simulink model "real_UIO_EEG_2021_03_03_01"  (R2019b)
settings: Solver=FixedStepAuto  StartTime=0.0  StopTime=180  FixedStep=0.01  RelTol=1e-3
values from neighbouring files (symbols this model uses):
  Am = double(subs(Am_sys,{ep,Lx},{0.1,1-2*j}))    [DAC_UIO_Comp.m]    (also in UIO_adaptive_example_EEG_Balas_2ch.m = [0 1;-5 -4]; UIO_adaptive_example_alternative_EEG_ch6.m = ss_c.A; UIO_alternative_2021_01_26.m = Am-.1*eye(2); UIO_alternative_PAPER_2021_02_17.m = [0 1;-1 -1])
  B = [0;1]    [DAC_UIO_Comp.m]    (also in UIO_adaptive_example_EEG_Balas_2ch.m; UIO_adaptive_example_alternative_EEG_ch6.m = ones(opt_order,1); UIO_alternative_2021_01_26.m; UIO_alternative_PAPER_2021_02_17.m = [1;0;-1])
  C = double(subs(C_sym,{ep},{0.1}))    [DAC_UIO_Comp.m]    (also in UIO_adaptive_example.m = [1 0 0 0 0;0 0 0 1 0; 0 0 0 0 1]; UIO_adaptive_example_2.m = [1 0 0 0;0 1 0 0]; UIO_adaptive_example_EEG_Balas_2ch.m = [1, epsilon]; UIO_adaptive_example_alternative_EEG_ch6.m = ss_c.C)
  Fu = mats    [UIO_adaptive_example_alternative_EEG_ch6.m]    (also in UIO_alternative_2021_01_26.m = [0 1 ;-25 0]; UIO_alternative_PAPER_2021_02_17.m = [0,0,0,0, 0;0 0 1 0 0;0 -25 0 0 0;0 0 0 0 1;0 0 0 -144 0]; UIO_alternative_PAPER_2021_03_01.m = [0 1 0 0;-25 0 0 0;0 0 0 1;0 0 -144 0]; UIO_alternative_PAPER_2021_03_02.m = [0 1 0 0;-25 0 0 0;0 0 0 1;0 0 -144 0])
  gamma_e = 1    [DAC_UIO_Comp.m]    (also in UIO_adaptive_example_EEG_Balas_2ch.m; UIO_adaptive_example_alternative_EEG_ch6.m = .0001*ones(length(Am),1); UIO_alternative_2021_01_26.m = 0.001; UIO_alternative_PAPER_2021_02_17.m = 0.0001)
  K1 = Klqr(1:length(Am),:)    [UIO_adaptive_example_alternative_EEG_ch6.m]    (also in UIO_alternative_PAPER_2021_03_02.m = Kout3(1:length(Am),:))
  K2 = Klqr(length(Am)+1:end,:)    [UIO_adaptive_example_alternative_EEG_ch6.m]    (also in UIO_alternative_PAPER_2021_03_02.m = Kout3(length(Am)+1:end,:))
  Theta = [real(Theta_cust);imag(Theta_cust)]    [LinearND_QUANTUM_2020_11_14_2.m]    (also in UIO_adaptive_example_alternative_EEG_ch6.m = ones(1,size(Fu,1)); UIO_alternative_2021_01_26.m = [1,1]; UIO_alternative_PAPER_2021_02_17.m = [1,1,1,1,1]; UIO_alternative_PAPER_2021_03_01.m = [1,1,1,1])
libraries: dspmtrx3 x1, simulink_extras x1
settings Model: Creator=Tris  LastModifiedBy=Tris
settings DataIOCC: ExternalInput="Y_sim1, Y_sim2, Y_sim3,  Y_sim4, Y_sim5, Y_sim6"  LoadExternalInput=on

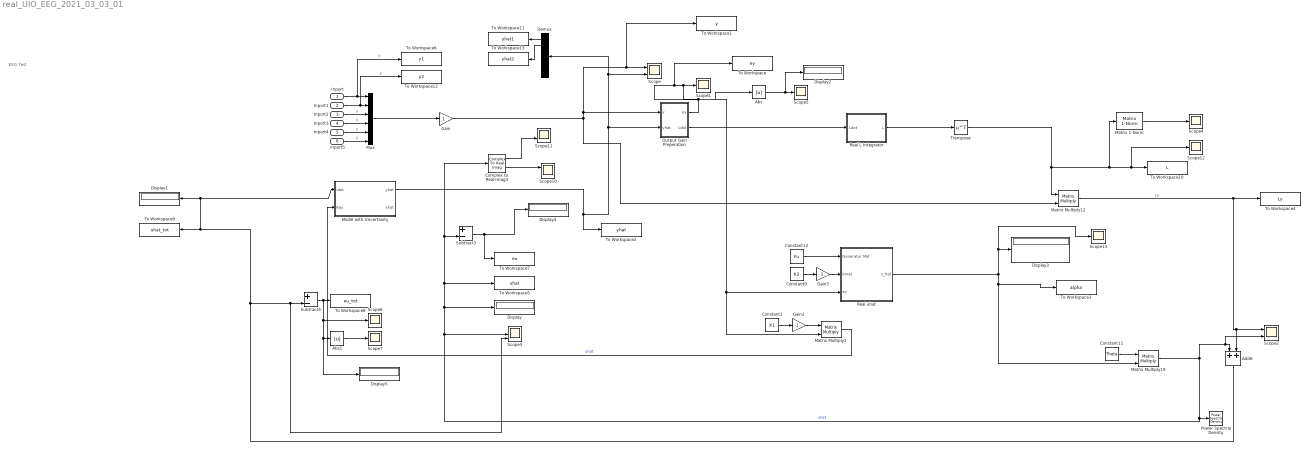
== system real_UIO_EEG_2021_03_03_01 ==
  note: EEG Test
  Inport : Inport
  Inport1 : Inport  Port=2
  Inport2 : Inport  Port=3
  Inport3 : Inport  Port=4
  Inport4 : Inport  Port=5
  Inport5 : Inport  Port=6
  Abs : Abs
  Abs1 : Abs
  Add6 : Sum
  Complex to Real-Imag3 : ComplexToRealImag
  Constant1 : Constant  Value=K1  VectorParams1D=off
  Constant11 : Constant  Value=Theta  VectorParams1D=off
  Constant12 : Constant  Value=Fu
  Constant9 : Constant  Value=K2  VectorParams1D=off
  Demux : Demux  Outputs=6
  Display{,1..5} (6 alike) : Display
  Gain : Gain
  Gain2 : Gain  Gain=-1
  Gain3 : Gain  Gain=-1
  Matrix 1-Norm : dspmtrx3/Matrix  1-Norm  roundingMode=Floor  overflowMode=off  outputDataTypeStr=Inherit: Same as accumulator  outputMin=[]  outputMax=[]  outputLastDataTypeStr=Inherit: Same as accumulator
      settings: SourceProductName=DSP System Toolbox  SourceProductBaseCode=DS
  Matrix Multiply1 : Product  Multiplication=Matrix(*)
  Matrix Multiply12 : Product  Multiplication=Matrix(*)
  Matrix Multiply19 : Product  Multiplication=Matrix(*)
  Model with Uncertainty : Subsystem
  Mux : Mux  Inputs=6
  Output Gain Preperation : Subsystem
  Power Spectral Density : simulink_extras/Additional Sinks/Power Spectral Density  npts=128  fftpts=512  HowOften=64  sampleT=0.1
      settings: SourceProductName=Simulink  SourceProductBaseCode=SL
  Real L Integrator : Subsystem
  "Real uhat " : Subsystem
  Scope{,2,10..11} (4 alike) : Scope  NumInputPorts=2
  Scope{1,4..7,12..13} (7 alike) : Scope
  Scope3 : Scope  NumInputPorts=3
  Subtract3 : Sum  Inputs=+-
  Subtract4 : Sum  Inputs=+-
  To Workspace : ToWorkspace  VariableName=ey  SaveFormat=Timeseries  SampleTime=-1
  To Workspace1 : ToWorkspace  VariableName=y  SaveFormat=Timeseries  SampleTime=-1
  To Workspace10 : ToWorkspace  VariableName=L  SaveFormat=Timeseries  SampleTime=-1
  To Workspace11 : ToWorkspace  VariableName=yhat1  SaveFormat=Timeseries  SampleTime=-1
  To Workspace12 : ToWorkspace  VariableName=y2  SaveFormat=Timeseries  SampleTime=-1
  To Workspace13 : ToWorkspace  VariableName=yhat2  SaveFormat=Timeseries  SampleTime=-1
  To Workspace2 : ToWorkspace  VariableName=yhat  SaveFormat=Timeseries  SampleTime=-1
  To Workspace3 : ToWorkspace  VariableName=alpha  SaveFormat=Timeseries  SampleTime=-1
  To Workspace4 : ToWorkspace  VariableName=Ly  SaveFormat=Timeseries  SampleTime=-1
  To Workspace5 : ToWorkspace  VariableName=uhat  SaveFormat=Timeseries  SampleTime=-1
  To Workspace6 : ToWorkspace  VariableName=y1  SaveFormat=Timeseries  SampleTime=-1
  To Workspace7 : ToWorkspace  VariableName=eu  SaveFormat=Timeseries  SampleTime=-1
  To Workspace8 : ToWorkspace  VariableName=eu_tot  SaveFormat=Timeseries  SampleTime=-1
  To Workspace9 : ToWorkspace  VariableName=uhat_tot  SaveFormat=Timeseries  SampleTime=-1
  Transpose : Math  Operator=transpose  SignedPower=off  SaturateOnIntegerOverflow=on
  wires:
  Constant11/1 -> Matrix Multiply19/1
  Matrix Multiply19/1 -> Add6/1, Scope2/2, Power Spectral Density/1, To Workspace5/1, Complex to Real-Imag3/1, Subtract3/2, Display/1, Scope3/2  "uhat"
  Matrix Multiply12/1 -> To Workspace4/1, Add6/2, Scope2/1  "Ly"
  Constant9/1 -> Gain3/1
  Constant12/1 -> "Real uhat "/1(Generator Mat)
  "Real uhat "/1(z_hat) -> To Workspace3/1, Matrix Multiply19/2, Scope13/1, Display3/1
  Real L Integrator/1(L) -> Transpose/1
  Abs/1 -> Display2/1, Scope5/1
  Model with Uncertainty/1(yhat) -> To Workspace2/1, Demux/1, Scope/2, Output Gain Preperation/2(yhat)
  Add6/1 -> Model with Uncertainty/1(utot), Display1/1, To Workspace9/1, Scope3/3, Subtract4/2
  Subtract3/1 -> Display4/1, To Workspace7/1
  Output Gain Preperation/2(Ldot) -> Real L Integrator/1(Ldot)
  Abs1/1 -> Scope7/1
  Complex to Real-Imag3/1 -> Scope11/2
  Complex to Real-Imag3/2 -> Scope10/1
  Subtract4/1 -> Display5/1, Abs1/1, Scope6/1, To Workspace8/1
  Matrix 1-Norm/1 -> Scope4/1
  Inport3/1 -> Mux/4  "y"
  Inport2/1 -> Mux/3  "y"
  Inport1/1 -> To Workspace12/1, Mux/2  "y"
  Inport5/1 -> Mux/6  "y"
  Inport4/1 -> Mux/5  "y"
  Gain3/1 -> "Real uhat "/2(Kmat)
  Gain2/1 -> Matrix Multiply1/1
  Constant1/1 -> Gain2/1
  Output Gain Preperation/1(ey) -> To Workspace/1, Abs/1, Scope1/1, Matrix Multiply1/2, "Real uhat "/3(ey)
  Matrix Multiply1/1 -> Model with Uncertainty/2(Key)  "uhat"
  Mux/1 -> Gain/1
  Gain/1 -> Matrix Multiply12/2, To Workspace1/1, Scope/1, Output Gain Preperation/1(y)
  Inport/1 -> To Workspace6/1, Mux/1  "y"
  Transpose/1 -> Matrix 1-Norm/1, Scope12/1, To Workspace10/1, Matrix Multiply12/1
  Demux/1 -> To Workspace11/1
  Demux/2 -> To Workspace13/1

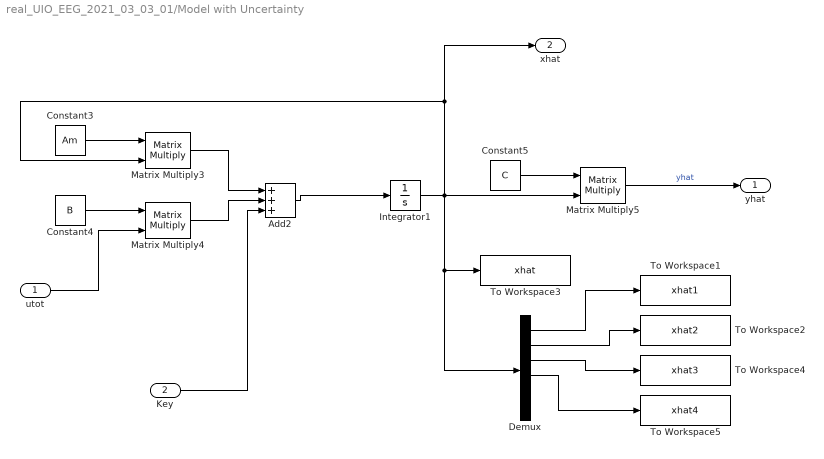
== system real_UIO_EEG_2021_03_03_01/Model with Uncertainty ==
  utot : Inport
  Key : Inport  Port=2
  Add2 : Sum  Inputs=+++
  Constant3 : Constant  Value=Am
  Constant4 : Constant  Value=B  VectorParams1D=off
  Constant5 : Constant  Value=C  VectorParams1D=off
  Demux : Demux  Outputs=6
  Integrator1 : Integrator
  Matrix Multiply3 : Product  Multiplication=Matrix(*)
  Matrix Multiply4 : Product  Multiplication=Matrix(*)
  Matrix Multiply5 : Product  Multiplication=Matrix(*)
  To Workspace1 : ToWorkspace  VariableName=xhat1  SaveFormat=Timeseries  SampleTime=-1
  To Workspace2 : ToWorkspace  VariableName=xhat2  SaveFormat=Timeseries  SampleTime=-1
  To Workspace3 : ToWorkspace  VariableName=xhat  SaveFormat=Timeseries  SampleTime=-1
  To Workspace4 : ToWorkspace  VariableName=xhat3  SaveFormat=Timeseries  SampleTime=-1
  To Workspace5 : ToWorkspace  VariableName=xhat4  SaveFormat=Timeseries  SampleTime=-1
  yhat : Outport
  xhat : Outport  Port=2
  wires:
  Constant3/1 -> Matrix Multiply3/1
  Integrator1/1 -> Demux/1, To Workspace3/1, Matrix Multiply5/2, xhat/1, Matrix Multiply3/2
  Constant5/1 -> Matrix Multiply5/1
  Add2/1 -> Integrator1/1
  Matrix Multiply4/1 -> Add2/2
  utot/1 -> Matrix Multiply4/2
  Constant4/1 -> Matrix Multiply4/1
  Matrix Multiply3/1 -> Add2/1
  Matrix Multiply5/1 -> yhat/1  "yhat"
  Key/1 -> Add2/3
  Demux/1 -> To Workspace1/1
  Demux/2 -> To Workspace2/1
  Demux/3 -> To Workspace4/1
  Demux/4 -> To Workspace5/1

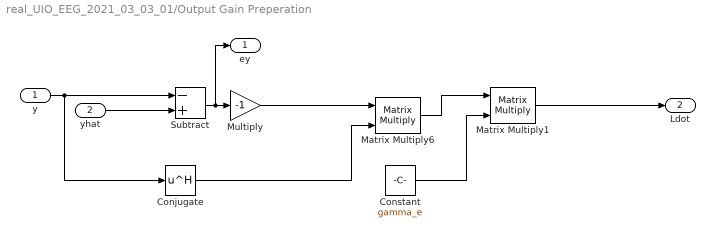
== system real_UIO_EEG_2021_03_03_01/Output Gain Preperation ==
  y : Inport
  yhat : Inport  Port=2
  Conjugate : Math  Operator=hermitian  RndMeth=Zero  SaturateOnIntegerOverflow=on
  Constant : Constant  Value=gamma_e  VectorParams1D=off
  Matrix Multiply1 : Product  Multiplication=Matrix(*)
  Matrix Multiply6 : Product  Multiplication=Matrix(*)
  Multiply : Gain  Gain=-1
  Subtract : Sum  Inputs=-+
  ey : Outport
  Ldot : Outport  Port=2
  wires:
  Matrix Multiply6/1 -> Matrix Multiply1/1
  Matrix Multiply1/1 -> Ldot/1
  Multiply/1 -> Matrix Multiply6/1
  y/1 -> Conjugate/1, Subtract/1
  yhat/1 -> Subtract/2
  Subtract/1 -> Multiply/1, ey/1
  Conjugate/1 -> Matrix Multiply6/2
  Constant/1 -> Matrix Multiply1/2

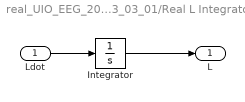
== system real_UIO_EEG_2021_03_03_01/Real L Integrator ==
  Ldot : Inport
  Integrator : Integrator
  L : Outport
  wires:
  Ldot/1 -> Integrator/1
  Integrator/1 -> L/1

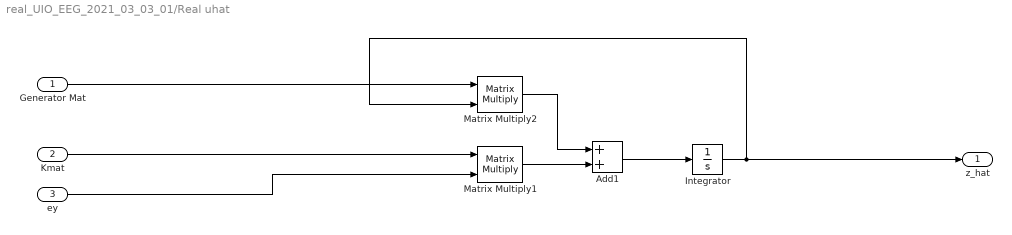
== system real_UIO_EEG_2021_03_03_01/Real uhat  ==
  Generator Mat : Inport
  Kmat : Inport  Port=2
  ey : Inport  Port=3
  Add1 : Sum
  Integrator : Integrator
  Matrix Multiply1 : Product  Multiplication=Matrix(*)
  Matrix Multiply2 : Product  Multiplication=Matrix(*)
  z_hat : Outport
  wires:
  ey/1 -> Matrix Multiply1/2
  Generator Mat/1 -> Matrix Multiply2/1
  Kmat/1 -> Matrix Multiply1/1
  Matrix Multiply1/1 -> Add1/2
  Add1/1 -> Integrator/1
  Matrix Multiply2/1 -> Add1/1
  Integrator/1 -> Matrix Multiply2/2, z_hat/1
